simulink model "PreLookup_kf_clip"  (R2017b)
settings: Solver=FixedStepAuto  StartTime=0.0  StopTime=10.0  FixedStep=0.1  RelTol=1e-3
settings Model: Creator=ktrinh  LastModifiedBy=hbourbou

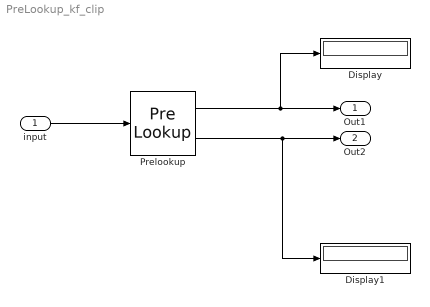
== system PreLookup_kf_clip ==
  input : Inport
  Display : Display
  Display1 : Display
  Prelookup : PreLookup  BreakpointsData=[10:10:110]
  Out1 : Outport
  Out2 : Outport  Port=2
  wires:
  input/1 -> Prelookup/1
  Prelookup/1 -> Display/1, Out1/1
  Prelookup/2 -> Display1/1, Out2/1
